simulink model "control3nema2"  (R2025b)
settings: Solver=FixedStepAuto  StartTime=0.0  StopTime=10.0  RelTol=1e-3  EnableMultiTasking=on
undefined symbols (not defined in the file): bits
libraries: stm32f4xxblockslib x9, simulink x6, stm32blockslib x6, svdutilitieslib x3
settings Model: STM32="{\"I2CControllerRead\":[{\"ID\":\"untitled1:33\"},{\"ID\":\"untitled1:86\"},{\"ID\":\"CONTROL2NEMA:33\"},{\"ID\":\"CONTROL2NEMA:86\"},{\"ID\":\"control3nema:245\"},{\"ID\":\"control3nema:33\"},{\"ID\":\"control3nema:86\"}],\"DigitalPortWrite\":[{\"ID\":\"untitled1:37\"},{\"ID\":\"untitled1:38\"},{\"ID\":\"untitled1:90\"},{\"ID\":\"untitled1:91\"},{\"ID\":\"CONTROL2NEMA:37\"},{\"ID\":\"CONTROL2NEMA:38\"},{\"ID\":\"CONTROL2NEMA:90\"},{\"ID\":\"CONTROL2NEMA:91\"},{\"ID\":\"control3nema:250\"},{\"ID\":\"control3nema:249\"},{\"ID\":\"control3nema:38\"},{\"ID\":\"control3nema:37\"},{\"ID\":\"control3nema:91\"},{\"ID\":\"control3nema:90\"}],\"PWMOutput\":[{\"ID\":\"untitled1:39\"},{\"ID\":\"untitled1:92\"},{\"ID\":\"CONTROL2NEMA:39\"},{\"ID\":\"CONTROL2NEMA:92\"},{\"ID\":\"control3nema:251\"},{\"ID\":\"control3nema:92\"},{\"ID\":\"control3nema:422\"}],\"UARTWrite\":[{\"ID\":\"untitled1:47\"},{\"ID\":\"untitled1:100\"},{\"ID\":\"CONTROL2NEMA:47\"},{\"ID\":\"CONTROL2NEMA:100\"},{\"ID\":\"control3nema:259\"},{\"ID\":\"control3nema:47\"},{\"ID\":\"control3nema:100\"}]}"  Creator=hnyur  LastModifiedBy=hnyur
settings OptimizationCC: DefaultParameterBehavior=Inlined  EnhancedBackFolding=on  PassReuseOutputArgsAs=Individual arguments  ZeroExternalMemoryAtStartup=off  ZeroInternalMemoryAtStartup=off  MaxStackSize=512  OptimizeBlockOrder=speed  DifferentSizesBufferReuse=on  OptimizationCustomize=off  EfficientTunableParamExpr=on
settings DebuggingCC: ParameterTunabilityLossMsg=error
settings HardwareCC: ProdBitPerPointer=32.0  ProdBitPerSizeT=32.0  ProdBitPerPtrDiffT=32.0  ProdLargestAtomicInteger=Long  ProdLargestAtomicFloat=Double  ProdWordSize=32.0  ProdLongLongMode=on  ProdHWDeviceType=ARM Compatible->ARM Cortex-M
settings SFSimCC: MATLABDynamicMemAlloc=off
settings RTWCC: SystemTargetFile=ert.tlc  HardwareBoard=STM32H7xx Based (Single-core)  TemplateMakefile=ert_default_tmf  Toolchain=GNU Tools for ARM Embedded Processors  Description=Embedded Coder
settings CodeAppCC: ForceParamTrailComments=on  IgnoreCustomStorageClasses=off  OperatorAnnotations=on  SimulinkDataObjDesc=on  SFDataObjDesc=on  InsertBlockDesc=on
settings ERTTargetCC: ExtModeTransport=3.0  ExtModeStaticAlloc=on  ExtModeStaticAllocSize=2048.0  ExtModeMexFile=ext_xcp  ExtModeIntrfLevel=Level2 - Open  TargetLangStandard=C99 (ISO)  CodeReplacementLibrary=ARM Cortex-M  SupportContinuousTime=on

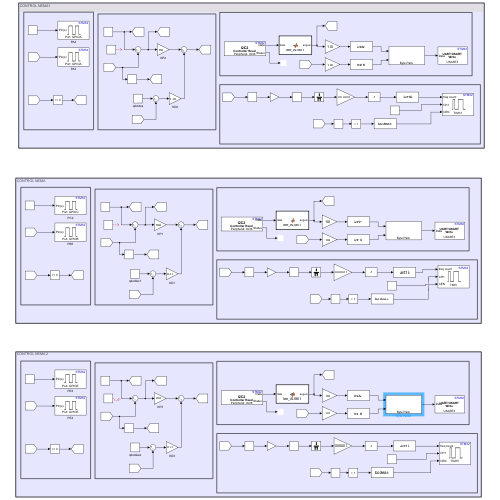
[thumbnail: Simulink's stored preview of the top-level diagram]
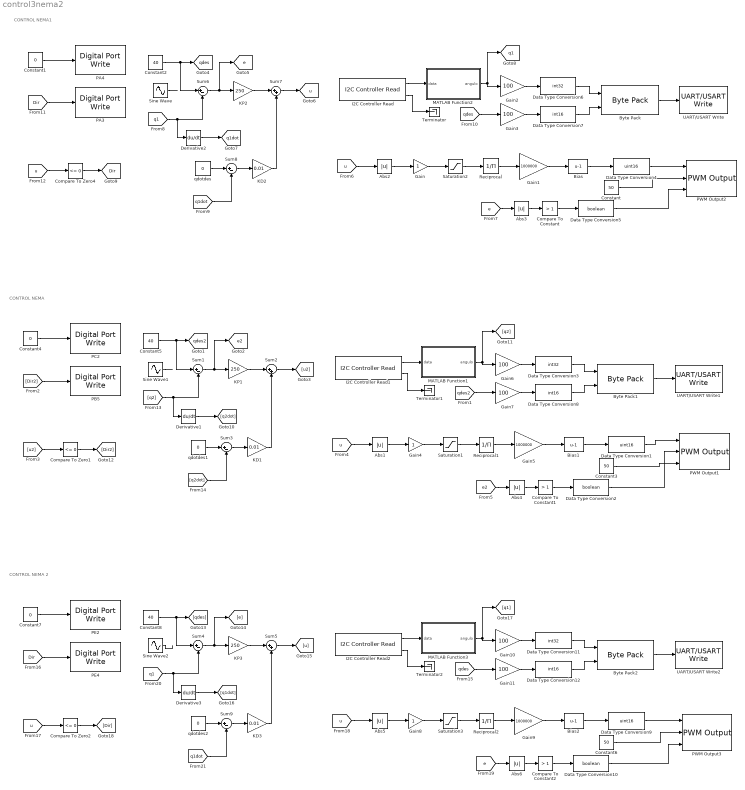
== system control3nema2 ==
  note: CONTROL NEMA 2
  note: CONTROL NEMA
  note: CONTROL NEMA1
  Abs{1..6} (6 alike) : Abs  SaturateOnIntegerOverflow=off
  Bias : Bias  Bias=-1  SaturateOnIntegerOverflow=off
  Bias1 : Bias  Bias=-1  SaturateOnIntegerOverflow=off
  Bias2 : Bias  Bias=-1  SaturateOnIntegerOverflow=off
  Byte Pack : svdutilitieslib/Byte Pack  maskPackedDataType=uint8  datatypes={'int32','int16'}  byteAlign=2  blockPlatform=tic2000
      settings: LibrarySourceBlock=c2000lib/Target Communication/Byte Pack
  Byte Pack1 : svdutilitieslib/Byte Pack  maskPackedDataType=uint8  datatypes={'int32','int16'}  byteAlign=2  blockPlatform=tic2000
      settings: LibrarySourceBlock=c2000lib/Target Communication/Byte Pack
  Byte Pack2 : svdutilitieslib/Byte Pack  maskPackedDataType=uint8  datatypes={'int32','int16'}  byteAlign=2  blockPlatform=tic2000
      settings: LibrarySourceBlock=c2000lib/Target Communication/Byte Pack
  Compare To Constant : simulink/Logic and Bit Operations/Compare To Constant  relop=>  const=1  OutDataTypeStr=boolean
  Compare To Constant1 : simulink/Logic and Bit Operations/Compare To Constant  relop=>  const=1  OutDataTypeStr=boolean
  Compare To Constant2 : simulink/Logic and Bit Operations/Compare To Constant  relop=>  const=1  OutDataTypeStr=boolean
  Compare To Zero1 : simulink/Logic and Bit Operations/Compare To Zero  relop=<=  OutDataTypeStr=boolean
  Compare To Zero2 : simulink/Logic and Bit Operations/Compare To Zero  relop=<=  OutDataTypeStr=boolean
  Compare To Zero4 : simulink/Logic and Bit Operations/Compare To Zero  relop=<=  OutDataTypeStr=boolean
  Constant : Constant  Value=50
  Constant1 : Constant  Value=0
  Constant2 : Constant  Value=40
  Constant3 : Constant  Value=50
  Constant4 : Constant  Value=0
  Constant5 : Constant  Value=40
  Constant6 : Constant  Value=50
  Constant7 : Constant  Value=0
  Constant8 : Constant  Value=40
  Data Type Conversion1 : DataTypeConversion  OutDataTypeStr=uint16  RndMeth=Floor
  Data Type Conversion10 : DataTypeConversion  OutDataTypeStr=boolean  RndMeth=Floor
  Data Type Conversion11 : DataTypeConversion  OutDataTypeStr=int32  SaturateOnIntegerOverflow=off  RndMeth=Floor
  Data Type Conversion12 : DataTypeConversion  OutDataTypeStr=int16  SaturateOnIntegerOverflow=off  RndMeth=Floor
  Data Type Conversion2 : DataTypeConversion  OutDataTypeStr=boolean  RndMeth=Floor
  Data Type Conversion3 : DataTypeConversion  OutDataTypeStr=int32  SaturateOnIntegerOverflow=off  RndMeth=Floor
  Data Type Conversion4 : DataTypeConversion  OutDataTypeStr=uint16  RndMeth=Floor
  Data Type Conversion5 : DataTypeConversion  OutDataTypeStr=boolean  RndMeth=Floor
  Data Type Conversion6 : DataTypeConversion  OutDataTypeStr=int32  SaturateOnIntegerOverflow=off  RndMeth=Floor
  Data Type Conversion7 : DataTypeConversion  OutDataTypeStr=int16  SaturateOnIntegerOverflow=off  RndMeth=Floor
  Data Type Conversion8 : DataTypeConversion  OutDataTypeStr=int16  SaturateOnIntegerOverflow=off  RndMeth=Floor
  Data Type Conversion9 : DataTypeConversion  OutDataTypeStr=uint16  RndMeth=Floor
  Derivative1 : Derivative
  Derivative2 : Derivative
  Derivative3 : Derivative  CoefficientInTFapproximation=0.001
  Gain : Gain
  Gain1 : Gain  Gain=1000000
  Gain{2..3,6..7,10..11} (6 alike) : Gain  Gain=100
  Gain4 : Gain
  Gain5 : Gain  Gain=1000000
  Gain8 : Gain
  Gain9 : Gain  Gain=1000000
  I2C Controller Read : stm32blockslib/I2C Controller Read  I2CModule=I2C2  Mode=Controller  AddressingMode=7-bits  PeripheralByteOrder=BigEndian  OwnPeripheralAddress=uint8(170)  PeripheralAddressVia=Dialog  PeripheralAddress=0x36  RegisterAddressMode=on  RegisterAddressVia=Dialog  RegisterAddress=14  RepeatedStart=off  NoAck=off  OutputStatus=on  BlockMode=Receive  DataType=uint8  DataLength=2  Timeout=0.001  SampleTime=0.001
      settings: LibrarySourceBlock=stm32h7xxblockslib/I2C Controller Read
  I2C Controller Read1 : stm32blockslib/I2C Controller Read  I2CModule=I2C2  Mode=Controller  AddressingMode=7-bits  PeripheralByteOrder=BigEndian  OwnPeripheralAddress=uint8(170)  PeripheralAddressVia=Dialog  PeripheralAddress=0x36  RegisterAddressMode=on  RegisterAddressVia=Dialog  RegisterAddress=14  RepeatedStart=off  NoAck=off  OutputStatus=on  BlockMode=Receive  DataType=uint8  DataLength=2  Timeout=0.001  SampleTime=0.001
      settings: LibrarySourceBlock=stm32h7xxblockslib/I2C Controller Read
  I2C Controller Read2 : stm32blockslib/I2C Controller Read  I2CModule=I2C2  Mode=Controller  AddressingMode=7-bits  PeripheralByteOrder=BigEndian  OwnPeripheralAddress=uint8(170)  PeripheralAddressVia=Dialog  PeripheralAddress=0x36  RegisterAddressMode=on  RegisterAddressVia=Dialog  RegisterAddress=14  RepeatedStart=off  NoAck=off  OutputStatus=on  BlockMode=Receive  DataType=uint8  DataLength=2  Timeout=0.001  SampleTime=0.001
      settings: LibrarySourceBlock=stm32h7xxblockslib/I2C Controller Read
  KD1 : Gain  Gain=0.01
  KD2 : Gain  Gain=0.01
  KD3 : Gain  Gain=0.01
  KP1 : Gain  Gain=250
  KP2 : Gain  Gain=250
  KP3 : Gain  Gain=250
  MATLAB Function1 : MATLAB Function  TreatAsAtomicUnit=on
  MATLAB Function2 : MATLAB Function  TreatAsAtomicUnit=on
  MATLAB Function3 : MATLAB Function  TreatAsAtomicUnit=on
  PA3 : stm32f4xxblockslib/Digital Port Write  PortName=GPIOA  PinNumber=3  ReadOperation=off  IOAsArray=on  EnableSimPort=off  hoistedMaskSrc=ECSoC/ECSimCodegen/Digital Port Write
      settings: LibrarySourceBlock=stm32h7xxblockslib/Digital Port Write
  PA4 : stm32f4xxblockslib/Digital Port Write  PortName=GPIOA  PinNumber=4  ReadOperation=off  IOAsArray=on  EnableSimPort=off  hoistedMaskSrc=ECSoC/ECSimCodegen/Digital Port Write
      settings: LibrarySourceBlock=stm32h7xxblockslib/Digital Port Write
  PB5 : stm32f4xxblockslib/Digital Port Write  PortName=GPIOB  PinNumber=5  ReadOperation=off  IOAsArray=on  EnableSimPort=off  hoistedMaskSrc=ECSoC/ECSimCodegen/Digital Port Write
      settings: LibrarySourceBlock=stm32h7xxblockslib/Digital Port Write
  PC2 : stm32f4xxblockslib/Digital Port Write  PortName=GPIOC  PinNumber=2  ReadOperation=off  IOAsArray=on  EnableSimPort=off  hoistedMaskSrc=ECSoC/ECSimCodegen/Digital Port Write
      settings: LibrarySourceBlock=stm32h7xxblockslib/Digital Port Write
  PE2 : stm32f4xxblockslib/Digital Port Write  PortName=GPIOE  PinNumber=2  ReadOperation=off  IOAsArray=on  EnableSimPort=off  hoistedMaskSrc=ECSoC/ECSimCodegen/Digital Port Write
      settings: LibrarySourceBlock=stm32h7xxblockslib/Digital Port Write
  PE4 : stm32f4xxblockslib/Digital Port Write  PortName=GPIOE  PinNumber=4  ReadOperation=off  IOAsArray=on  EnableSimPort=off  hoistedMaskSrc=ECSoC/ECSimCodegen/Digital Port Write
      settings: LibrarySourceBlock=stm32h7xxblockslib/Digital Port Write
  PWM Output1 : stm32f4xxblockslib/PWM Output  ProcessorFamily=STM32G4  TimerModule=TIM3  DutycycleUnits=Counts  EnableChannel1=on  EnableCaptureCompare1Input=off  EnableCaptureCompare1ComplementaryInput=off  EnableOutputCompare1ModeInput=off  EnableChannel2=off  EnableCaptureCompare2Input=off  EnableCaptureCompare2ComplementaryInput=off  EnableOutputCompare2ModeInput=off  EnableChannel3=off  EnableCaptureCompare3Input=off  EnableCaptureCompare3ComplementaryInput=off  EnableOutputCompare3ModeInput=off  EnableChannel4=off  EnableCaptureCompare4Input=off  EnableCaptureCompare4ComplementaryInput=off  EnableOutputCompare4ModeInput=off  EnableChannel5=off  EnableCaptureCompare5Input=off  EnableOutputCompare5ModeInput=off  EnableChannel6=off  EnableCaptureCompare6Input=off  EnableOutputCompare6ModeInput=off  EnableCounterInput=on  EnableMainOutputInput=off  EnableFrequencyInput=on  SetRCAfterCE=off  OutputDirection=off  OutputMainOutputEnableStatus=off  SampleTime=0.1  EnableSimPort=off  EnableUpdateEvent=off  EnableCaptureCompare1Event=off  EnableCaptureCompare2Event=off  EnableCaptureCompare3Event=off  EnableCaptureCompare4Event=off  EnableTriggerEvent=off  EnableBreakEvent=off  EnableBreakEvent2=off  hoistedMaskSrc=ECSoC/ECSimCodegen/PWM Output
      settings: LibrarySourceBlock=stm32h7xxblockslib/PWM Output
  PWM Output2 : stm32f4xxblockslib/PWM Output  ProcessorFamily=STM32G4  TimerModule=TIM13  DutycycleUnits=Counts  EnableChannel1=on  EnableCaptureCompare1Input=off  EnableCaptureCompare1ComplementaryInput=off  EnableOutputCompare1ModeInput=off  EnableChannel2=on  EnableCaptureCompare2Input=off  EnableCaptureCompare2ComplementaryInput=off  EnableOutputCompare2ModeInput=off  EnableChannel3=on  EnableCaptureCompare3Input=off  EnableCaptureCompare3ComplementaryInput=off  EnableOutputCompare3ModeInput=off  EnableChannel4=off  EnableCaptureCompare4Input=off  EnableCaptureCompare4ComplementaryInput=off  EnableOutputCompare4ModeInput=off  EnableChannel5=off  EnableCaptureCompare5Input=off  EnableOutputCompare5ModeInput=off  EnableChannel6=off  EnableCaptureCompare6Input=off  EnableOutputCompare6ModeInput=off  EnableCounterInput=on  EnableMainOutputInput=off  EnableFrequencyInput=on  SetRCAfterCE=off  OutputDirection=off  OutputMainOutputEnableStatus=off  SampleTime=0.1  EnableSimPort=off  EnableUpdateEvent=off  EnableCaptureCompare1Event=off  EnableCaptureCompare2Event=off  EnableCaptureCompare3Event=off  EnableCaptureCompare4Event=off  EnableTriggerEvent=off  EnableBreakEvent=off  EnableBreakEvent2=off  hoistedMaskSrc=ECSoC/ECSimCodegen/PWM Output
      settings: LibrarySourceBlock=stm32h7xxblockslib/PWM Output
  PWM Output3 : stm32f4xxblockslib/PWM Output  ProcessorFamily=STM32G4  TimerModule=TIM15  DutycycleUnits=Counts  EnableChannel1=on  EnableCaptureCompare1Input=off  EnableCaptureCompare1ComplementaryInput=off  EnableOutputCompare1ModeInput=off  EnableChannel2=off  EnableCaptureCompare2Input=off  EnableCaptureCompare2ComplementaryInput=off  EnableOutputCompare2ModeInput=off  EnableChannel3=off  EnableCaptureCompare3Input=off  EnableCaptureCompare3ComplementaryInput=off  EnableOutputCompare3ModeInput=off  EnableChannel4=off  EnableCaptureCompare4Input=off  EnableCaptureCompare4ComplementaryInput=off  EnableOutputCompare4ModeInput=off  EnableChannel5=off  EnableCaptureCompare5Input=off  EnableOutputCompare5ModeInput=off  EnableChannel6=off  EnableCaptureCompare6Input=off  EnableOutputCompare6ModeInput=off  EnableCounterInput=on  EnableMainOutputInput=off  EnableFrequencyInput=on  SetRCAfterCE=off  OutputDirection=off  OutputMainOutputEnableStatus=off  SampleTime=0.1  EnableSimPort=off  EnableUpdateEvent=off  EnableCaptureCompare1Event=off  EnableCaptureCompare2Event=off  EnableCaptureCompare3Event=off  EnableCaptureCompare4Event=off  EnableTriggerEvent=off  EnableBreakEvent=off  EnableBreakEvent2=off  hoistedMaskSrc=ECSoC/ECSimCodegen/PWM Output
      settings: LibrarySourceBlock=stm32h7xxblockslib/PWM Output
  Reciprocal : Product  Inputs=/
  Reciprocal1 : Product  Inputs=/
  Reciprocal2 : Product  Inputs=/
  Saturation1 : Saturate  UpperLimit=8000  LowerLimit=1
  Saturation2 : Saturate  UpperLimit=8000  LowerLimit=1
  Saturation3 : Saturate  UpperLimit=8000  LowerLimit=1
  Sine Wave : Sin  Amplitude=180  SampleTime=0.001
  Sine Wave1 : Sin  Amplitude=180  SampleTime=0.001
  Sine Wave2 : Sin  Amplitude=180  SampleTime=0.001
  Sum{1,3..4,6,8..9} (6 alike) : Sum  Inputs=|+-
  Sum2 : Sum  Inputs=|++
  Sum5 : Sum  Inputs=|++
  Sum7 : Sum  Inputs=|++
  Terminator : Terminator
  Terminator1 : Terminator
  Terminator2 : Terminator
  UART/USART Write : stm32blockslib/UART//USART Write  UARTModule=USART3  LengthOfDataToSend=off  BlockingMode=off  BlockingTimeout=0.1  OutputStatus=off
      settings: LibrarySourceBlock=stm32h7xxblockslib/UART//USART Write
  UART/USART Write1 : stm32blockslib/UART//USART Write  UARTModule=USART3  LengthOfDataToSend=off  BlockingMode=off  BlockingTimeout=0.1  OutputStatus=off
      settings: LibrarySourceBlock=stm32h7xxblockslib/UART//USART Write
  UART/USART Write2 : stm32blockslib/UART//USART Write  UARTModule=USART3  LengthOfDataToSend=off  BlockingMode=off  BlockingTimeout=0.1  OutputStatus=off
      settings: LibrarySourceBlock=stm32h7xxblockslib/UART//USART Write
  qdotdes : Constant  Value=0
  qdotdes1 : Constant  Value=0
  qdotdes2 : Constant  Value=0
  tag scope: Dir=global, e2=global, e=global, q1=global, q1dot=global, qdes2=global, qdes=global, u=global
  wires:
  [Dir] -> PA3/1
  Reciprocal/1 -> Gain1/1
  [e] -> Abs3/1
  [qdes] -> Gain3/1
  Sum7/1 -> [u]
  Constant1/1 -> PA4/1
  KP2/1 -> Sum7/1
  Sine Wave/1 -> ?
  [q1dot] -> Sum8/2
  Abs2/1 -> Gain/1
  Compare To Zero4/1 -> [Dir]
  Saturation2/1 -> Reciprocal/1
  Gain1/1 -> Bias/1
  Bias/1 -> Data Type Conversion4/1
  KD2/1 -> Sum7/2
  Gain/1 -> Saturation2/1
  Compare To Constant/1 -> Data Type Conversion5/1
  Data Type Conversion4/1 -> PWM Output2/1
  Sum6/1 -> KP2/1, [e]
  qdotdes/1 -> Sum8/1
  Data Type Conversion6/1 -> Byte Pack/1
  Constant/1 -> PWM Output2/2
  [u] -> Abs2/1
  Gain2/1 -> Data Type Conversion6/1
  [q1] -> Sum6/2, Derivative2/1
  Sum8/1 -> KD2/1
  Gain3/1 -> Data Type Conversion7/1
  Data Type Conversion7/1 -> Byte Pack/2
  MATLAB Function2/1(angulo) -> Gain2/1, [q1]
  Byte Pack/1 -> UART/USART Write/1
  I2C Controller Read/1 -> MATLAB Function2/1(data)
  Abs3/1 -> Compare To Constant/1
  [u] -> Compare To Zero4/1
  I2C Controller Read/2 -> Terminator/1
  Constant2/1 -> Sum6/1, [qdes]
  Derivative2/1 -> [q1dot]
  Data Type Conversion5/1 -> PWM Output2/3
  Data Type Conversion2/1 -> PWM Output1/2
  Derivative1/1 -> [q2dot]
  Constant5/1 -> [qdes2], Sum1/1
  I2C Controller Read1/2 -> Terminator1/1
  [u2] -> Compare To Zero1/1
  Abs4/1 -> Compare To Constant1/1
  I2C Controller Read1/1 -> MATLAB Function1/1(data)
  Byte Pack1/1 -> UART/USART Write1/1
  MATLAB Function1/1(angulo) -> [q2], Gain6/1
  Data Type Conversion8/1 -> Byte Pack1/2
  Gain7/1 -> Data Type Conversion8/1
  Sum3/1 -> KD1/1
  [q2] -> Derivative1/1, Sum1/2
  Gain6/1 -> Data Type Conversion3/1
  [u] -> Abs1/1
  Constant3/1 -> PWM Output1/3
  Data Type Conversion3/1 -> Byte Pack1/1
  qdotdes1/1 -> Sum3/1
  Sum1/1 -> [e2], KP1/1
  Data Type Conversion1/1 -> PWM Output1/1
  Compare To Constant1/1 -> Data Type Conversion2/1
  Gain4/1 -> Saturation1/1
  KD1/1 -> Sum2/2
  Bias1/1 -> Data Type Conversion1/1
  Gain5/1 -> Bias1/1
  Saturation1/1 -> Reciprocal1/1
  Compare To Zero1/1 -> [Dir2]
  Abs1/1 -> Gain4/1
  [q2dot] -> Sum3/2
  Sine Wave1/1 -> ?
  KP1/1 -> Sum2/1
  Constant4/1 -> PC2/1
  Sum2/1 -> [u2]
  [qdes2] -> Gain7/1
  [e2] -> Abs4/1
  Reciprocal1/1 -> Gain5/1
  [Dir2] -> PB5/1
  Data Type Conversion10/1 -> PWM Output3/3
  Derivative3/1 -> [q1dot]
  Constant8/1 -> [qdes], Sum4/1
  I2C Controller Read2/2 -> Terminator2/1
  [u] -> Compare To Zero2/1
  Abs6/1 -> Compare To Constant2/1
  I2C Controller Read2/1 -> MATLAB Function3/1(data)
  Byte Pack2/1 -> UART/USART Write2/1
  MATLAB Function3/1(angulo) -> [q1], Gain10/1
  Data Type Conversion12/1 -> Byte Pack2/2
  Gain11/1 -> Data Type Conversion12/1
  Sum9/1 -> KD3/1
  [q1] -> Derivative3/1, Sum4/2
  Gain10/1 -> Data Type Conversion11/1
  [u] -> Abs5/1
  Constant6/1 -> PWM Output3/2
  Data Type Conversion11/1 -> Byte Pack2/1
  qdotdes2/1 -> Sum9/1
  Sum4/1 -> [e], KP3/1
  Data Type Conversion9/1 -> PWM Output3/1
  Compare To Constant2/1 -> Data Type Conversion10/1
  Gain8/1 -> Saturation3/1
  KD3/1 -> Sum5/2
  Bias2/1 -> Data Type Conversion9/1
  Gain9/1 -> Bias2/1
  Saturation3/1 -> Reciprocal2/1
  Compare To Zero2/1 -> [Dir]
  Abs5/1 -> Gain8/1
  [q1dot] -> Sum9/2
  Sine Wave2/1 -> ?
  KP3/1 -> Sum5/1
  Constant7/1 -> PE2/1
  Sum5/1 -> [u]
  [qdes] -> Gain11/1
  [e] -> Abs6/1
  Reciprocal2/1 -> Gain9/1
  [Dir] -> PE4/1

== matlab function control3nema2/MATLAB Function2 ==
  data: data input; angulo output
function angulo = leer_AS5600(data)
% Variables persistentes:
% angulo_anterior almacena la ultima lectura del sensor.
% posicion acumula la posicion angular relativa.
persistent angulo_anterior posicion
% Separar los dos bytes recibidos mediante I2C.
byte_alto = uint16(data(1));
byte_bajo = uint16(data(2));
% Reconstruir el valor de 12 bits del encoder.
conteo = bitor(bitshift(byte_alto,8), byte_bajo);
% Eliminar los cuatro bits que no contienen informacion.
conteo = bitand(conteo,uint16(4095));
% Convertir el conteo a grados.
angulo_actual = double(conteo)*360.0/4096.0;

% Inicializacion de las variables persistentes.
if isempty(angulo_anterior)
angulo_anterior = angulo_actual;
posicion = 0.0;
end
% Calcular el desplazamiento angular entre muestras.
delta = angulo_actual- angulo_anterior;
% Corregir el cambio entre 359 grados y 0 grados.
if delta > 180.0
delta = delta- 360.0;
elseif delta <-180.0
delta = delta + 360.0;
end
% Acumular la posicion relativa.
posicion = posicion + delta;
% Actualizar la lectura anterior.
angulo_anterior = angulo_actual;
% Devolver la posicion angular.
angulo = posicion;
end

== matlab function control3nema2/MATLAB Function1 ==
  data: data input; angulo output
function angulo = leer_AS5600(data)
% Variables persistentes:
% angulo_anterior almacena la ultima lectura del sensor.
% posicion acumula la posicion angular relativa.
persistent angulo_anterior posicion
% Separar los dos bytes recibidos mediante I2C.
byte_alto = uint16(data(1));
byte_bajo = uint16(data(2));
% Reconstruir el valor de 12 bits del encoder.
conteo = bitor(bitshift(byte_alto,8), byte_bajo);
% Eliminar los cuatro bits que no contienen informacion.
conteo = bitand(conteo,uint16(4095));
% Convertir el conteo a grados.
angulo_actual = double(conteo)*360.0/4096.0;

% Inicializacion de las variables persistentes.
if isempty(angulo_anterior)
angulo_anterior = angulo_actual;
posicion = 0.0;
end
% Calcular el desplazamiento angular entre muestras.
delta = angulo_actual- angulo_anterior;
% Corregir el cambio entre 359 grados y 0 grados.
if delta > 180.0
delta = delta- 360.0;
elseif delta <-180.0
delta = delta + 360.0;
end
% Acumular la posicion relativa.
posicion = posicion + delta;
% Actualizar la lectura anterior.
angulo_anterior = angulo_actual;
% Devolver la posicion angular.
angulo = posicion;
end

== matlab function control3nema2/MATLAB Function3 ==
  data: data input; angulo output
function angulo = leer_AS5600(data)
% Variables persistentes:
% angulo_anterior almacena la ultima lectura del sensor.
% posicion acumula la posicion angular relativa.
persistent angulo_anterior posicion
% Separar los dos bytes recibidos mediante I2C.
byte_alto = uint16(data(1));
byte_bajo = uint16(data(2));
% Reconstruir el valor de 12 bits del encoder.
conteo = bitor(bitshift(byte_alto,8), byte_bajo);
% Eliminar los cuatro bits que no contienen informacion.
conteo = bitand(conteo,uint16(4095));
% Convertir el conteo a grados.
angulo_actual = double(conteo)*360.0/4096.0;

% Inicializacion de las variables persistentes.
if isempty(angulo_anterior)
angulo_anterior = angulo_actual;
posicion = 0.0;
end
% Calcular el desplazamiento angular entre muestras.
delta = angulo_actual- angulo_anterior;
% Corregir el cambio entre 359 grados y 0 grados.
if delta > 180.0
delta = delta- 360.0;
elseif delta <-180.0
delta = delta + 360.0;
end
% Acumular la posicion relativa.
posicion = posicion + delta;
% Actualizar la lectura anterior.
angulo_anterior = angulo_actual;
% Devolver la posicion angular.
angulo = posicion;
end
